simulink subsystem "PieroBel_Model_z"  (R2023b)
settings: Solver=VariableStepAuto  StartTime=0.0  StopTime=10.0  RelTol=1e-3
settings Model: Creator=marqu  LastModifiedBy=marqu

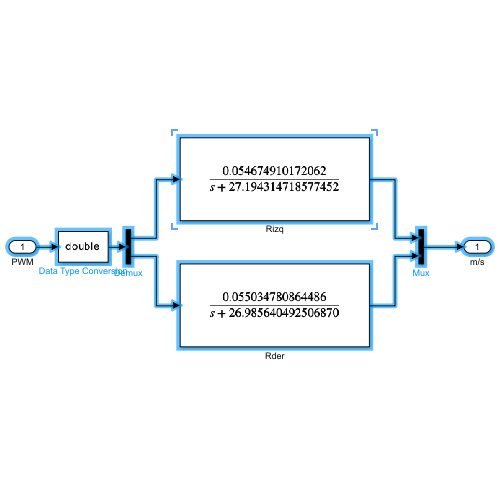
[thumbnail: Simulink's stored preview of the top-level diagram]
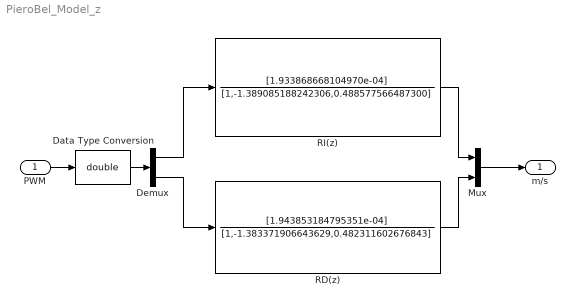
== system PieroBel_Model_z ==
  PWM : Inport
  Data Type Conversion : DataTypeConversion  OutDataTypeStr=double  SaturateOnIntegerOverflow=off  RndMeth=Floor
  Demux : Demux  Outputs=2
  Mux : Mux  Inputs=2
  RD(z) : DiscreteFilter  Numerator=[1.943853184795351e-04]  Denominator=[1,-1.383371906643629,0.482311602676843]
  RI(z) : DiscreteFilter  Numerator=[1.933868668104970e-04]  Denominator=[1,-1.389085188242306,0.488577566487300]
  m/s : Outport
  wires:
  PWM/1 -> Data Type Conversion/1
  Data Type Conversion/1 -> Demux/1
  Mux/1 -> m/s/1
  Demux/2 -> RD(z)/1
  Demux/1 -> RI(z)/1
  RD(z)/1 -> Mux/2
  RI(z)/1 -> Mux/1
